simulink model "Simulink_Filtro_valor_mas_alto"  (R2018b)
settings: Solver=VariableStepAuto  StartTime=0.0  StopTime=10.0  RelTol=1e-3
libraries: dspstat3 x2, dspsnks4 x1, dspsrcs4 x1
settings Model: Creator=alexa  LastModifiedBy=alexa

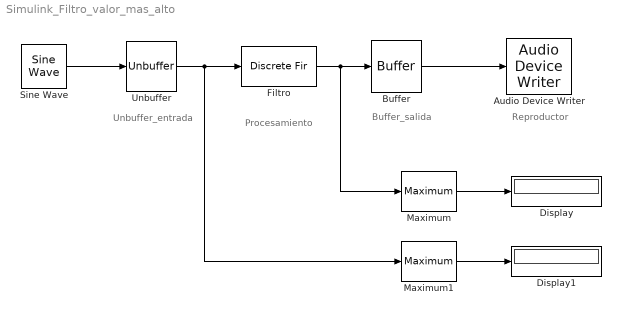
== system Simulink_Filtro_valor_mas_alto ==
  note: Procesamiento
  note: Unbuffer_entrada
  note: Buffer_salida
  note: Reproductor
  Audio Device Writer : dspsnks4/Audio Device Writer  Driver=DirectSound  Device=Default  InheritSampleRate=on  SampleRate=44100  BitDepth=16-bit integer  BufferSize=4096  NumBuffers=10  DefaultOutputChannelMapping=on  OutputChannelMapping=1:2  OutputNumUnderrunSamples=off  DriverIdx=1  DeviceWarnFlag=''
  Buffer : Buffer  OutputFrames=off
  Display : Display
  Display1 : Display
  Filtro : DiscreteFir  Tag=BlockMethodSubSystem  Coefficients=[0.000192222707916954661 0.000309219800150138484 0.000422005901286501197 0.000529581846294212332 0.000631004652221989638 0.000725398396577585803 0.000811964437746644577 0.000889990851918536483 0.000958860968432039169 0.00101806089436112779 0.00106718592944590176 0.00110594578403453835 0.0011341685254226898 0.00115180319172456273 0.00115892102704004537 0.00115571530703697969 0.00114249973997937351 0.00111970544452461886 0.0010878765221022785 0.00104766425818675975 0.000999820003095218748 0.000945186798890405746 0.000884689834357103616 0.000819325824665259345 0.000750151426054935155 0.000678270808507579702 0.000604822520744609628 0.000530965791871391697 0.000457866422428572235 0.000386682424406478719 0.000318549574822071888 0.000254567050670873778 0.000195783314387376395 0.000143182418336737944 9.7670894299793282e-05 6.0065389406212457e-05 3.10812035434312377e-05 1.13218749702691053e-05 1.26995076429951533e-06 1.27906692372434418e-06 1.15674495401831744e-05 3.22129335915990979e-05 6.31495797247592743e-05 0.000104165952074042301 0.000154905101878799202 0.000214866282614077539 0.000283408402745580993 0.000359755202276911706 0.000443002119198954701 0.000532124792005459943 0.000625989124835060122 0.000723362822766448251 0.000822928286555649332 0.000923296738880349474 0.00102302343815686655 0.00112062382141904135 0.0012145904047802436 0.00130341025880917447 0.00138558286688852928 0.00145963816742400768 0.00152415457573912391 0.00157777677871492991 0.0016192330947755369 0.00164735219371537852 0.00166107897512362125 0.00165948941076758129 0.00164180416520730657 0.0016074008200573542 0.00155582454059289698 0.0014867970386937704 0.00140022370328581492 0.00129619878830448108 0.00117500856858069507 0.00103713239572312686 0.000883241608816709607 0.000714196278332061667 0.000531039785788945925 0.000334991266174698688 0.000127435964613343969 -9.00864169624909062e-05 -0.000315895283643383368 -0.000548184499433375036 -0.000785039382859929052 -0.00102445518139076749 -0.00126435684073870273 -0.00150261986793275427 -0.00173709207185161621 -0.00196561595195154535 -0.00218605149535062602 -0.00239629913440548258 -0.00259432261155970352 -0.00277817149565062933 -0.00294600309410009576 -0.0030961035085194516 -0.00322690758723438113 -0.00333701753705219597 -0.00342521996819308535 -0.00349050116059514831 -0.00353206035665744669 -0.00354932090475250546 -0.00354193909933689464 -0.00350981058700618924 -0.00345307423314404355 -0.00337211337064612137 -0.00326755438028068432 -0.00314026258128243451 -0.00299133544045542595 -0.00282209313806263198 -0.00263406655877581729 -0.00242898280561562683 -0.00220874836379589485 -0.00197543006936598282 -0.00173123406419802808 -0.00147848294387816393 -0.00121959132813321538 -0.000957040104275650436 -0.000693349612517809807 -0.000431052057656517167 -0.000172663444349464731 7.93446571840287449e-05 0.000322573201852013284 0.000554723300602096405 0.000773623075861079763 0.000977253429770792931 0.00116377242095141087 0.00133153795644997503 0.00147912851985024262 0.00160536167411935975 0.00170931009849986095 0.00179031494243814238 0.00184799630595390281 0.00188226068474867223 0.00189330524944312942 0.00188161886131410451 0.00184797976143876233 0.00179344990589115172 0.00171936595620191023 0.00162732697129990217 0.00151917888420803138 0.00139699588346346758 0.00126305885517135914 0.00111983107638125522 0.000969931383704244099 0.000816105072384712936 0.000661192810039850417 0.000508097875636288952 0.000359752057666995007 0.000219080565628614933 8.89663255188904496e-05 -2.77859570527200628e-05 -0.000128485573609683448 -0.000210591032024931308 -0.000271744320168269696 -0.000309803819546254308 -0.000322875482378555964 -0.000309341897693094533 -0.000267888888344984576 -0.00019752930125630896 -9.76236774735753777e-05 3.21024833559964144e-05 0.00019154511802608917 0.000380211873632860318 0.00059721644207408873 0.000841277097026366192 0.00111071953315808867 0.001403484063562584 0.00171713718636843857 0.00204888748565941947 ...(+8203 chars)]  InputProcessing=Columns as channels (frame based)
  Maximum : dspstat3/Maximum  operation=maximum  fcn=Value  indexBase=One  operateOver=Entire input  Dimension=1  InputProcessing=Columns as channels (frame based)  reset=None  roiEnable=off  roiType=Rectangles  roiPortion=Entire ROI  roiOutput=Individual statistics for each ROI  roiFlag=off  roundingMode=Floor  overflowMode=off  accumDataTypeStr=Inherit: Same as product output  accumLastDataTypeStr=Inherit: Same as product output
  Maximum1 : dspstat3/Maximum  operation=maximum  fcn=Value  indexBase=One  operateOver=Entire input  Dimension=1  InputProcessing=Columns as channels (frame based)  reset=None  roiEnable=off  roiType=Rectangles  roiPortion=Entire ROI  roiOutput=Individual statistics for each ROI  roiFlag=off  roundingMode=Floor  overflowMode=off  accumDataTypeStr=Inherit: Same as product output  accumLastDataTypeStr=Inherit: Same as product output
  Sine Wave : dspsrcs4/Sine Wave  Amplitude=1  Frequency=1000  Phase=0  SampleMode=Discrete  OutComplex=Real  CompMethod=Trigonometric fcn  TableSize=Speed  SampleTime=1/44100  SamplesPerFrame=1  ResetState=Restart at time zero  OutputFrames=off  dataType=double  wordLen=16  udDataType=sfix(16)  fracBitsMode=Best precision  numFracBits=15  OutDataTypeStr=double  LastOutDataTypeStr=double
  Unbuffer : Unbuffer
  wires:
  Buffer/1 -> Audio Device Writer/1
  Filtro/1 -> Maximum/1, Buffer/1
  Sine Wave/1 -> Unbuffer/1
  Unbuffer/1 -> Maximum1/1, Filtro/1
  Maximum1/1 -> Display1/1
  Maximum/1 -> Display/1
